simulink model "GenPT001"  (Simulink 8.3)
settings: Solver=ode45  StartTime=0.0  StopTime=10.0  RelTol=1e-3
model workspace (MAT data in the model file):
  Trans.transRatio = 22.5
  Engine : struct (value not decoded)
settings Model: Creator=swami  LastModifiedBy=swami
settings DataIOCC: SignalLoggingSaveFormat=Dataset
settings DebuggingCC: UnderspecifiedInitializationDetection=Simplified  StateNameClashWarn=none
settings GRTTargetCC: CombineOutputUpdateFcns=on  GRTInterface=off

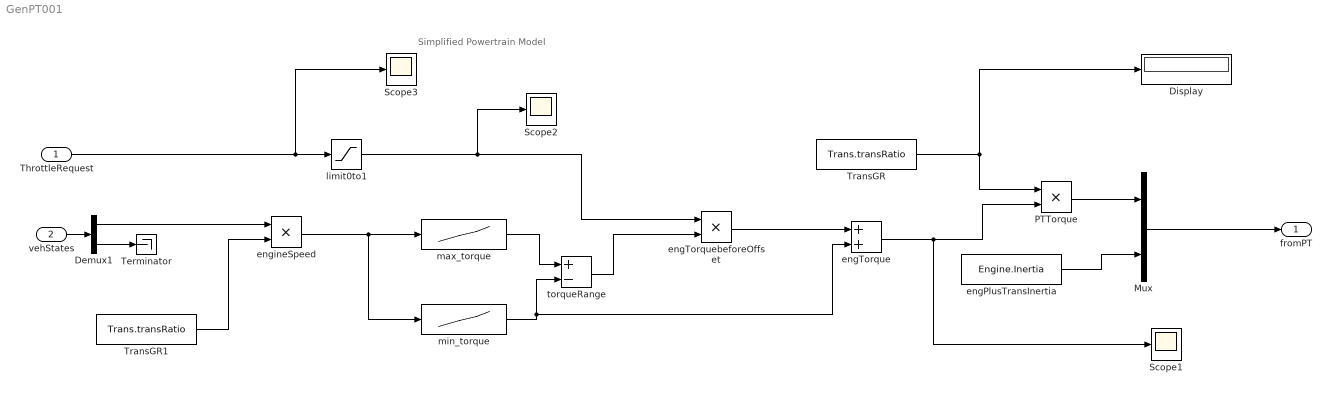
== system GenPT001 ==
  note: Simplified Powertrain Model
  ThrottleRequest : Inport
  vehStates : Inport  Port=2  PortDimensions=2
  Demux1 : Demux  Outputs=2
  Display : Display
  Mux : Mux  Inputs=2
  PTTorque : Product  Inputs=**
  Scope1 : Scope
  Scope2 : Scope
      settings: SaveName=ScopeData2
  Scope3 : Scope
      settings: SaveName=ScopeData3
  Terminator : Terminator
  TransGR : Constant  Value=Trans.transRatio
  TransGR1 : Constant  Value=Trans.transRatio
  engPlusTransInertia : Constant  Value=Engine.Inertia
  engTorque : Sum
  engTorquebeforeOffset : Product  Inputs=**
  engineSpeed : Product  Inputs=**
  limit0to1 : Saturate  UpperLimit=1  LowerLimit=0
  max_torque : Lookup_n-D  NumberOfTableDimensions=1  BreakpointsForDimension1=[0,60,70,600]  Table=[0, 0,150,150]  InternalRulePriority=Speed  RndMeth=Simplest  InputSameDT=on
  min_torque : Lookup_n-D  NumberOfTableDimensions=1  BreakpointsForDimension1=[0,600]  Table=[0, 0]  InternalRulePriority=Speed  RndMeth=Simplest  InputSameDT=on
  torqueRange : Sum  Inputs=+-
  fromPT : Outport
  wires:
  Mux/1 -> fromPT/1
  vehStates/1 -> Demux1/1
  ThrottleRequest/1 -> Scope3/1, limit0to1/1
  max_torque/1 -> torqueRange/1
  min_torque/1 -> engTorque/2, torqueRange/2
  torqueRange/1 -> engTorquebeforeOffset/2
  limit0to1/1 -> Scope2/1, engTorquebeforeOffset/1
  TransGR/1 -> PTTorque/1, Display/1
  PTTorque/1 -> Mux/1
  engPlusTransInertia/1 -> Mux/2
  Demux1/2 -> Terminator/1
  TransGR1/1 -> engineSpeed/2
  Demux1/1 -> engineSpeed/1
  engineSpeed/1 -> min_torque/1, max_torque/1
  engTorquebeforeOffset/1 -> engTorque/1
  engTorque/1 -> Scope1/1, PTTorque/2
